simulink library "M5Core_TestLibrary"  (R2023a)
settings: Solver=VariableStepAuto  StartTime=0.0  StopTime=10.0  RelTol=1e-3
undefined symbols (not defined in the file or in its folder): gain
libraries: simulink x9, hdlsllib x3
settings Model: Creator=auw_a  LastModifiedBy=auw_a

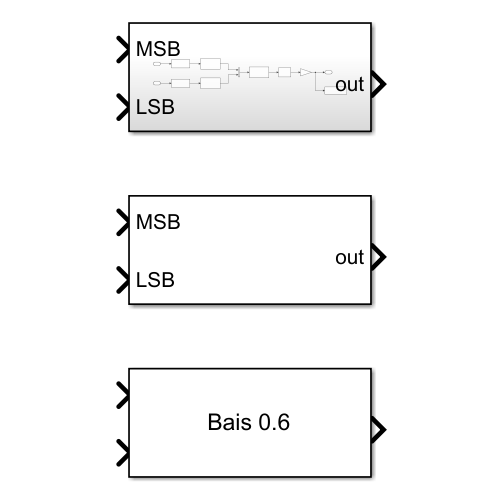
[thumbnail: Simulink's stored preview of the top-level diagram]
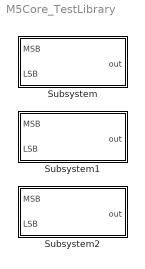
== system M5Core_TestLibrary ==
  Subsystem : Subsystem
  Subsystem1 : Subsystem  mask{gain=0.25}
      mask prompts: gain "Enter Bais Value"
  Subsystem2 : Subsystem  mask{gain=.6}
      mask prompts: gain "Enter Bais Value"
      mask init:
      | str = "Bais " + gain;
      | label = str;
      mask Display: disp(label);

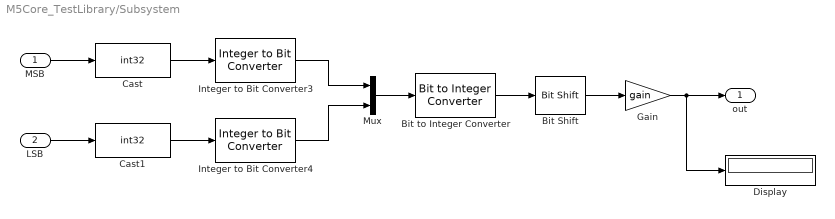
== system M5Core_TestLibrary/Subsystem ==
  MSB : Inport
  LSB : Inport  Port=2
  Bit Shift : hdlsllib/Logic and Bit Operations/Bit Shift  mode=Shift Right Logical  N=3
  Bit to Integer Converter : simulink/Logic and Bit Operations/Bit to Integer Converter  nbits=16  bitOrder=MSB first  signedOutputValues=Unsigned  outDtype=Inherit via internal rule  outDtypeSigned=Inherit via internal rule
  Cast : DataTypeConversion  OutDataTypeStr=int32  SaturateOnIntegerOverflow=off  RndMeth=Floor
  Cast1 : DataTypeConversion  OutDataTypeStr=int32  SaturateOnIntegerOverflow=off  RndMeth=Floor
  Display : Display
  Gain : Gain  Gain=gain
  Integer to Bit Converter3 : simulink/Logic and Bit Operations/Integer to Bit Converter  nbits=8  signedInputValues=Unsigned  bitOrder=MSB first  outDtype=Same as input
  Integer to Bit Converter4 : simulink/Logic and Bit Operations/Integer to Bit Converter  nbits=8  signedInputValues=Unsigned  bitOrder=MSB first  outDtype=Same as input
  Mux : Mux  Inputs=2
  out : Outport
  wires:
  LSB/1 -> Cast1/1
  Cast1/1 -> Integer to Bit Converter4/1
  Cast/1 -> Integer to Bit Converter3/1
  MSB/1 -> Cast/1
  Gain/1 -> out/1, Display/1
  Mux/1 -> Bit to Integer Converter/1
  Integer to Bit Converter3/1 -> Mux/1
  Bit Shift/1 -> Gain/1
  Bit to Integer Converter/1 -> Bit Shift/1
  Integer to Bit Converter4/1 -> Mux/2

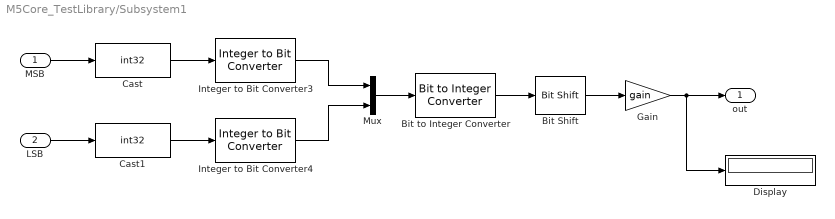
== system M5Core_TestLibrary/Subsystem1 ==
  MSB : Inport
  LSB : Inport  Port=2
  Bit Shift : hdlsllib/Logic and Bit Operations/Bit Shift  mode=Shift Right Logical  N=3
  Bit to Integer Converter : simulink/Logic and Bit Operations/Bit to Integer Converter  nbits=16  bitOrder=MSB first  signedOutputValues=Unsigned  outDtype=Inherit via internal rule  outDtypeSigned=Inherit via internal rule
  Cast : DataTypeConversion  OutDataTypeStr=int32  SaturateOnIntegerOverflow=off  RndMeth=Floor
  Cast1 : DataTypeConversion  OutDataTypeStr=int32  SaturateOnIntegerOverflow=off  RndMeth=Floor
  Display : Display
  Gain : Gain  Gain=gain
  Integer to Bit Converter3 : simulink/Logic and Bit Operations/Integer to Bit Converter  nbits=8  signedInputValues=Unsigned  bitOrder=MSB first  outDtype=Same as input
  Integer to Bit Converter4 : simulink/Logic and Bit Operations/Integer to Bit Converter  nbits=8  signedInputValues=Unsigned  bitOrder=MSB first  outDtype=Same as input
  Mux : Mux  Inputs=2
  out : Outport
  wires:
  LSB/1 -> Cast1/1
  Cast1/1 -> Integer to Bit Converter4/1
  Cast/1 -> Integer to Bit Converter3/1
  MSB/1 -> Cast/1
  Gain/1 -> out/1, Display/1
  Mux/1 -> Bit to Integer Converter/1
  Integer to Bit Converter3/1 -> Mux/1
  Bit Shift/1 -> Gain/1
  Bit to Integer Converter/1 -> Bit Shift/1
  Integer to Bit Converter4/1 -> Mux/2

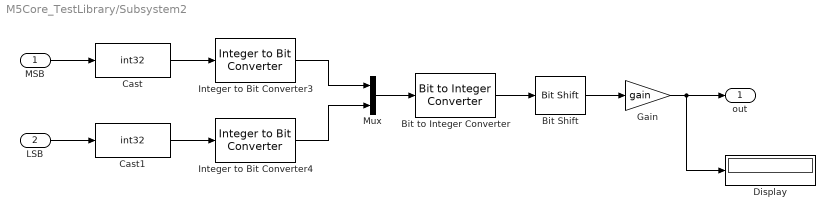
== system M5Core_TestLibrary/Subsystem2 ==
  MSB : Inport
  LSB : Inport  Port=2
  Bit Shift : hdlsllib/Logic and Bit Operations/Bit Shift  mode=Shift Right Logical  N=3
  Bit to Integer Converter : simulink/Logic and Bit Operations/Bit to Integer Converter  nbits=16  bitOrder=MSB first  signedOutputValues=Unsigned  outDtype=Inherit via internal rule  outDtypeSigned=Inherit via internal rule
  Cast : DataTypeConversion  OutDataTypeStr=int32  SaturateOnIntegerOverflow=off  RndMeth=Floor
  Cast1 : DataTypeConversion  OutDataTypeStr=int32  SaturateOnIntegerOverflow=off  RndMeth=Floor
  Display : Display
  Gain : Gain  Gain=gain
  Integer to Bit Converter3 : simulink/Logic and Bit Operations/Integer to Bit Converter  nbits=8  signedInputValues=Unsigned  bitOrder=MSB first  outDtype=Same as input
  Integer to Bit Converter4 : simulink/Logic and Bit Operations/Integer to Bit Converter  nbits=8  signedInputValues=Unsigned  bitOrder=MSB first  outDtype=Same as input
  Mux : Mux  Inputs=2
  out : Outport
  wires:
  LSB/1 -> Cast1/1
  Cast1/1 -> Integer to Bit Converter4/1
  Cast/1 -> Integer to Bit Converter3/1
  MSB/1 -> Cast/1
  Gain/1 -> out/1, Display/1
  Mux/1 -> Bit to Integer Converter/1
  Integer to Bit Converter3/1 -> Mux/1
  Bit Shift/1 -> Gain/1
  Bit to Integer Converter/1 -> Bit Shift/1
  Integer to Bit Converter4/1 -> Mux/2
